simulink model "RC_sim"  (R2022b)
settings: Solver=VariableStepDiscrete  StartTime=0.0  StopTime=100  FixedStep=1e-3  MaxStep=1e-3  RelTol=1e-3
undefined symbols (not defined in the file or in its folder): DiscIntNeverNeededParam
settings Model: Creator=brbar  LastModifiedBy=brbar

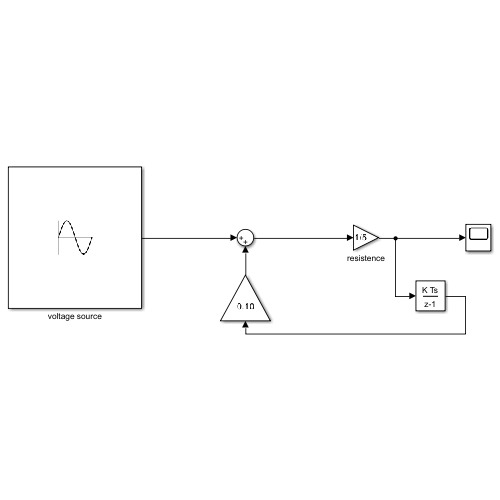
[thumbnail: Simulink's stored preview of the top-level diagram]
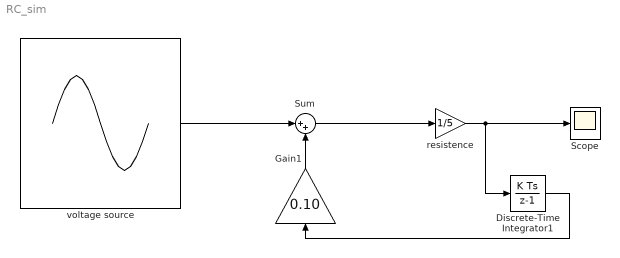
== system RC_sim ==
  Discrete-Time Integrator1 : DiscreteIntegrator  SampleTime=-1  ICPrevOutput=DiscIntNeverNeededParam  ICPrevScaledInput=DiscIntNeverNeededParam
  Gain1 : Gain  Gain=0.10
  Scope : Scope
  Sum : Sum  Inputs=|++
  resistence : Gain  Gain=1/5
  voltage source : Sin  SampleTime=0
  wires:
  voltage source/1 -> Sum/1
  Sum/1 -> resistence/1
  resistence/1 -> Discrete-Time Integrator1/1, Scope/1
  Discrete-Time Integrator1/1 -> Gain1/1
  Gain1/1 -> Sum/2
